simulink model "EOM"  (R2020a)
settings: Solver=VariableStepAuto  StartTime=0.0  StopTime=10.0  RelTol=1e-3
undefined symbols (not defined in the file): factstruct, ft, Hermes_2, m, s
libraries: aerolibconvert2 x3, shared6dof x1, aerolibadyn x1, aerolibatmos2 x1
settings Model: Creator=Shaan Heugly  LastModifiedBy=Shaan Heugly

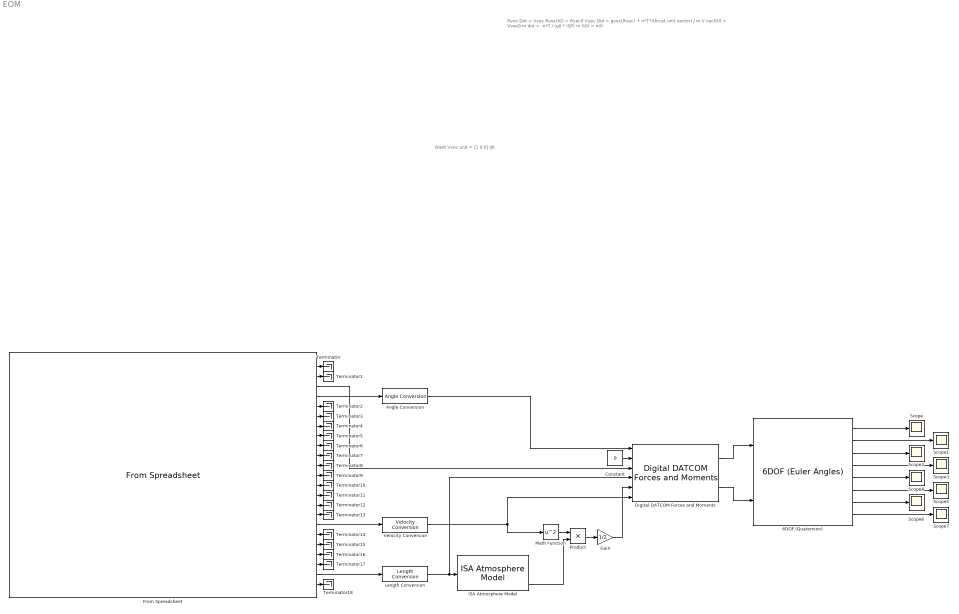
== system EOM ==
  note: Want Vvec unit = [1 0 0] IJK
  note: Rvec Dot = Vvec Rvec(t0) = Rvec0
      | Vvec Dot = gvec(Rvec) + n*T*(thrust unit vector) / m V vec(t0) = Vvec0
      | m dot = -n*T / (g0 * ISP) m (t0) = m0
  6DOF (Quaternion) : shared6dof/6DOF (Euler Angles)  units=Metric (MKS)  mtype=Fixed  rep=Quaternion  xme_0=[0 0 0]  Vm_0=[0 0 0]  eul_0=[0 0 0]  pm_0=[0 0 0]  mass_0=1.0  mass_e=0.5  mass_f=2.0  inertia=eye(3)  inertia_e=eye(3)  inertia_f=2*eye(3)  k_quat=1.0  vre_flag=on  abi_flag=off  aMode=0  xme_statename=''  Vm_statename=''  eul_statename=''  quat_statename=''  pm_statename=''  mass_statename=''
      settings: SourceProductBaseCode=AE,PW,MT,VE,VP
  Angle Conversion : aerolibconvert2/Angle Conversion  IU=deg  OU=rad
  Constant : Constant  Value=0
  Digital DATCOM Forces and Moments : aerolibadyn/Digital DATCOM Forces and Moments  units=Metric (MKS)  dcase=factstruct{1}  fmode=Body  buildno=0  imethod=None - flat  emethod=None - clip  rmethod=Clip to Range  action=None
      settings: SourceProductBaseCode=AE
  From Spreadsheet : FromSpreadsheet  FileName=D:\A.1 Documents\OneDrive\Documents\MATLAB\AE 403 Coding\px4Simuink\Shaan's Shit\Hermes_2-3_Flight_Data.xls  SheetName=Hermes_2-3_Flight_Data
  Gain : Gain  Gain=1/2
  ISA Atmosphere Model : aerolibatmos2/ISA Atmosphere Model  custom=off  g=9.80665  gamma=1.4  R=287.0531  L=0.0065  h_trop=11000  h_strat=20000  rho0=1.225  P0=101325  T0=288.15  h0=0
  Length Conversion : aerolibconvert2/Length Conversion  IU=ft  OU=m
  Math Function : Math  Operator=square  SaturateOnIntegerOverflow=on
  Product : Product
  Scope{,1..7} (8 alike) : Scope
  Terminator{,1..18} (19 alike) : Terminator
  Velocity Conversion : aerolibconvert2/Velocity Conversion  IU=ft/s  OU=m/s
  wires:
  Digital DATCOM Forces and Moments/1 -> 6DOF (Quaternion)/1
  Digital DATCOM Forces and Moments/2 -> 6DOF (Quaternion)/2
  From Spreadsheet/3 -> Digital DATCOM Forces and Moments/3
  From Spreadsheet/17 -> Velocity Conversion/1
  From Spreadsheet/4 -> Angle Conversion/1
  Angle Conversion/1 -> Digital DATCOM Forces and Moments/1
  From Spreadsheet/22 -> Length Conversion/1
  Length Conversion/1 -> Digital DATCOM Forces and Moments/4, ISA Atmosphere Model/1
  Velocity Conversion/1 -> Digital DATCOM Forces and Moments/6, Math Function/1
  ISA Atmosphere Model/4 -> Product/2
  Math Function/1 -> Product/1
  Product/1 -> Gain/1
  Gain/1 -> Digital DATCOM Forces and Moments/5
  Constant/1 -> Digital DATCOM Forces and Moments/2
  From Spreadsheet/5 -> Terminator2/1
  From Spreadsheet/6 -> Terminator3/1
  From Spreadsheet/7 -> Terminator4/1
  From Spreadsheet/8 -> Terminator5/1
  From Spreadsheet/9 -> Terminator6/1
  From Spreadsheet/10 -> Terminator7/1
  From Spreadsheet/11 -> Terminator8/1
  From Spreadsheet/12 -> Terminator9/1
  From Spreadsheet/13 -> Terminator10/1
  From Spreadsheet/14 -> Terminator11/1
  From Spreadsheet/15 -> Terminator12/1
  From Spreadsheet/16 -> Terminator13/1
  From Spreadsheet/18 -> Terminator14/1
  From Spreadsheet/19 -> Terminator15/1
  From Spreadsheet/20 -> Terminator16/1
  From Spreadsheet/21 -> Terminator17/1
  From Spreadsheet/23 -> Terminator18/1
  From Spreadsheet/1 -> Terminator/1
  From Spreadsheet/2 -> Terminator1/1
  6DOF (Quaternion)/1 -> Scope/1
  6DOF (Quaternion)/2 -> Scope1/1
  6DOF (Quaternion)/3 -> Scope2/1
  6DOF (Quaternion)/4 -> Scope3/1
  6DOF (Quaternion)/5 -> Scope4/1
  6DOF (Quaternion)/6 -> Scope5/1
  6DOF (Quaternion)/7 -> Scope6/1
  6DOF (Quaternion)/8 -> Scope7/1
